simulink model "ARDroneHover"  (R2019a)
settings: Solver=ode1  StartTime=0.0  StopTime=inf  FixedStep=sampleTime  RelTol=1e-3  EnableMultiTasking=on
values from neighbouring files (symbols this model uses):
  choice = input('')    [setupTT.m]
  K = lqr(A,B,Q,R)    [setupTT.m]
  k_w = 1    [setupTT.m]
  sampleTime = 0.03    [setupTT.m]
undefined symbols (not defined in the file or in its folder): DiscIntNeverNeededParam, Standard_Devices, UDP_Protocol
libraries: hdlsllib x6, dspnetwork x4, sldrtlib x3, simulink x1
(part 2 of 2)

== matlab function ARDroneHover/Outer-loop Controller/Error Scopes/normalize angle between -pi and pi radians ==
  data: angleIn input; angleOut output
function angleOut = fcn(angleIn)
%#codegen

angleOut = mod(angleIn, 2*pi) ;
if angleOut > pi
    angleOut = -2*pi + angleOut ; 
end

== matlab function ARDroneHover/Outer-loop Controller/MATLAB Function ==
  data: w_r output; dot_psi_r output; theta_r output; states input; pd input; dot_pd input; ddot_pd input; psi_d input; xi input; phi_r output; dot_xi output; k_w input; K input
function [w_r, dot_psi_r, theta_r, phi_r, dot_xi] = tt_controller(states, pd, dot_pd, ddot_pd,psi_d,xi, k_w, K)
%#codegen

% ------------------------------------------------------------------------
% inputs:
% states - structure with state variables
% pd - desired position
% dot_pd - desired velocity
% ddot_pt - desired acceleration
% psi_d - desired yaw angle
% xi - integral state (four variables)
%
% outputs:
% w_r - vertical velocity reference
% dot_psi_r - yaw rate reference
% theta_r - pitch angle reference
% phi_r - roll angle reference
% dot_xi - integral state derivative
% ------------------------------------------------------------------------

lambda      = states(1:3,1); % Euler angles
psi         = lambda(3);
R           = euler2R(lambda);
Rz          = [cos(psi) -sin(psi) 0; sin(psi) cos(psi) 0; 0 0 1];
psi_e       = normalize_angle(psi-psi_d);

p           = states(7:9,1); % position vector
p(3)        = p(3); % height is symmetric of z
vb          = states(4:6,1); % velocity vector in body coordinates
dot_p       = R*vb; % body velocity rotated to inertial frame 
dot_p(3)    = dot_p(3);

%!!!!!!!!!!!!!!!!!!!!!!!!!!!!!!!!!!!!!!!!!!!!!!!!!!!!!!!!!!!!!!!!!!!!!!
% replace with the necessary code to implement the trajectory tracking
% controller
% pd(3)       = pd(3);
% dot_pd(3)   = dot_pd(3);

% HEIGHT CONTROL
w_r     = -k_w*(p(3) - pd(3));

% OTHER CONTROL
tilde_x     = [p - pd; dot_p - dot_pd];

u_star      = Rz^(-1)*(K*tilde_x + [0; 0; 9.81] - ddot_pd + xi(1:3));

k_w         = 0;
theta_r     = atan(u_star(1)/u_star(3));
phi_r       = atan(-u_star(2)/sqrt(u_star(1)^2+u_star(3)^2));
dot_xi      = [k_w*1*K*tilde_x; psi_e];
dot_xi(3)   = dot_xi(3);

% PSI CONTROL
dot_psi_r   = -1*psi_e - 0.1*xi(4);
%!!!!!!!!!!!!!!!!!!!!!!!!!!!!!!!!!!!!!!!!!!!!!!!!!!!!!!!!!!!!!!!!!!!!!!


function R = euler2R(l)
%#codegen
% returns the rotation matrix for a given vector of euler angles

phi = l(1); theta = l(2); psi = l(3);
R = [cos(theta)*cos(psi)...
      sin(phi)*sin(theta)*cos(psi)-cos(phi)*sin(psi)...
      cos(phi)*sin(theta)*cos(psi)+sin(phi)*sin(psi);
   cos(theta)*sin(psi)...
   sin(phi)*sin(theta)*sin(psi)+cos(phi)*cos(psi)... 
   cos(phi)*sin(theta)*sin(psi)-sin(phi)*cos(psi);
   -sin(theta)...
   sin(phi)*cos(theta)...
   cos(phi)*cos(theta)];

function angleOut = normalize_angle(angleIn)
%#codegen

angleOut = mod(angleIn, 2*pi) ;
if angleOut > pi
    angleOut = -2*pi + angleOut ; 
end

== matlab function ARDroneHover/Data to States/Compute the Derivative/MATLAB Function ==
  data: u input; y output
function y = ZOH_nan(u)

persistent u_

if isempty(u_)
    u_ = 0;
end

if isnan(u)
    u = u_;
else
    u_ = u;
end

y = u;

== matlab function ARDroneHover/Data to States/Compute the Derivative/MATLAB Function1 ==
  data: u input; y output
function y = ZOH_nan(u)

persistent u_

if isempty(u_)
    u_ = 0;
end

if isnan(u)
    u = u_;
else
    u_ = u;
end

y = u;

== matlab function ARDroneHover/Data to States/Compute the Derivative/MATLAB Function2 ==
  data: u input; y output
function y = ZOH_nan(u)

persistent u_

if isempty(u_)
    u_ = 0;
end

if isnan(u)
    u = u_;
else
    u_ = u;
end

y = u;

== matlab function ARDroneHover/Data from Qualisys/Subsystem/MATLAB Function1 ==
  data: x4 output uint8; x3 output uint8; x2 output uint8; data input; x1 output uint8; object input
function [x4,x3,x2,x1] = fcn(data,object)

slot=(object-1)*8;

x1=data(41+slot);
x2=data(41+slot+1);
x3=data(41+slot+2);
x4=data(41+slot+3);

== matlab function ARDroneHover/Data from Qualisys/Subsystem/MATLAB Function2 ==
  data: x input uint32 size=1; X output single size=1; y input; Y output; z input; roll input; pitch input; yaw input; Z output; Roll output; Pitch output; Yaw output
function [X,Y,Z,Roll,Pitch,Yaw] = fcn(x,y,z,roll,pitch,yaw)


X = typecast(uint32(x),'single');
Y = typecast(uint32(y),'single');
Z = typecast(uint32(z),'single');
Roll = typecast(uint32(roll),'single');
Pitch = typecast(uint32(pitch),'single');
Yaw = typecast(uint32(yaw),'single');

== matlab function ARDroneHover/Data from Qualisys/Subsystem/MATLAB Function3 ==
  data: y4 output uint8; y3 output uint8; y2 output uint8; data input; y1 output uint8; object input
function [y4,y3,y2,y1] = fcn(data,object)

slot=(object-1)*8;

y1=data(45+slot);
y2=data(45+slot+1);
y3=data(45+slot+2);
y4=data(45+slot+3);

== matlab function ARDroneHover/Data from Qualisys/Subsystem/MATLAB Function4 ==
  data: z4 output uint8; z3 output uint8; z2 output uint8; data input; z1 output uint8; object input
function [z4,z3,z2,z1] = fcn(data,object)

slot=(object-1)*8;

z1=data(49+slot);
z2=data(49+slot+1);
z3=data(49+slot+2);
z4=data(49+slot+3);

== matlab function ARDroneHover/Data from Qualisys/Subsystem/MATLAB Function5 ==
  data: roll4 output uint8; roll3 output uint8; roll2 output uint8; data input; roll1 output uint8; object input
function [roll4,roll3,roll2,roll1] = fcn(data,object)

slot=(object-1)*8;

roll1=data(53+slot);
roll2=data(53+slot+1);
roll3=data(53+slot+2);
roll4=data(53+slot+3);

== matlab function ARDroneHover/Data from Qualisys/Subsystem/MATLAB Function6 ==
  data: pitch4 output uint8; pitch3 output uint8; pitch2 output uint8; data input; pitch1 output uint8; object input
function [pitch4,pitch3,pitch2,pitch1] = fcn(data,object)

slot=(object-1)*8;

pitch1=data(57+slot);
pitch2=data(57+slot+1);
pitch3=data(57+slot+2);
pitch4=data(57+slot+3);

== matlab function ARDroneHover/Data from Qualisys/Subsystem/MATLAB Function7 ==
  data: yaw4 output uint8; yaw3 output uint8; yaw2 output uint8; data input; yaw1 output uint8; object input
function [yaw4,yaw3,yaw2,yaw1] = fcn(data,object)

slot=(object-1)*8;

yaw1=data(61+slot);
yaw2=data(61+slot+1);
yaw3=data(61+slot+2);
yaw4=data(61+slot+3);

== matlab function ARDroneHover/Data to States/MATLAB Function ==
  data: v input; v_b output; phi input; theta input; psi input
function v_b = fcn(v,phi,theta,psi)

R = [cos(theta)*cos(psi)...
      sin(phi)*sin(theta)*cos(psi)-cos(phi)*sin(psi)...
      cos(phi)*sin(theta)*cos(psi)+sin(phi)*sin(psi);
   cos(theta)*sin(psi)...
   sin(phi)*sin(theta)*sin(psi)+cos(phi)*cos(psi)... 
   cos(phi)*sin(theta)*sin(psi)-sin(phi)*cos(psi);
   -sin(theta)...
   sin(phi)*cos(theta)...
   cos(phi)*cos(theta)];

v_b = R'*v;

== matlab function ARDroneHover/MATLAB Function1 ==
  data: on_off input; states input; t input; pd output; dot_pd output; ddot_pd output; psi_d output; choice input
function [pd, dot_pd, ddot_pd, psi_d] = desired_trajectory(on_off,states,t, choice)
%#codegen

% ------------------------------------------------------------------------
% inputs:
% on_off - 1 if tracking is on, 0 if it is off
% states - structure with state variables
% t - current simulation time
% 
% outputs:
% pd - desired position
% dot_pd - desired velocity
% ddot_pd - desired acceleration
% psi_d - desired yaw angle
% ------------------------------------------------------------------------

persistent t0
persistent p0
persistent previous_status

on  = 1;
off = 0;

BASE_ALT = 1;

% RESETS THE 0
if isempty(previous_status)
    previous_status = on;
    p0 = [states(7:8);BASE_ALT];
end

if on_off == off
    if previous_status == on 
    % first time off or switching back off
        p0 = [states(7:8);BASE_ALT]; % x0 and y0 match the current position
    end
    pd = p0;
    dot_pd = [0;0;0];
    ddot_pd = [0;0;0];
    psi_d = 0;
else
    if isempty(t0) || (previous_status == off) 
    % first time on or switching back on
        t0 = t;
        p0 = [states(7:8);BASE_ALT];
    end
    dt = t-t0;

%!!!!!!!!!!!!!!!!!!!!!!!!!!!!!!!!!!!!!!!!!!!!!!!!!!!!!!!!!!!!!!!!!!!!!!!!
% replace with the necessary code to define adequate desired trajectories
% use dt, p0, and any additional parameters

pd      = p0;
t_init  = 10;
t_track = 20;

% DEFINES THE STARTING HEIGHT
if(dt > t_init)
    pd(3) = pd(3) + 0.25;  
else
    pd(3) = pd(3) + 0;  
end

% DIFFERENT TRACKS
switch choice
    %--- Altitude Tracking ---
    case 1
      dot_pd    = [0;0;0];
      ddot_pd   = [0;0;0];
      psi_d     = 0;
    % --- Horizontal Line in X-Y ---
    case 2
      ang = 45;
      vel = 0.5;

      if(dt > t_track)
        dot_pd  = [vel*cosd(ang); vel*sind(ang);0];
        pd(1)   = p0(1) + vel*cosd(ang)*(dt - t_track);
        pd(2)   = p0(2) + vel*sind(ang)*(dt - t_track);
      else
        dot_pd  = [0;0;0]; 
      end
      
      ddot_pd   = [0;0;0];
      psi_d     = 0;
    % --- Circular Line - Constant Yaw ---
	case 3
      ang_rate = 0.1; %rad/s

      if(dt > t_track)
        pd(1:2)	= [ cos(ang_rate*(dt - t_track)) - 1;... 
                    sin(ang_rate*(dt - t_track))];
        dot_pd	= [-sin(ang_rate*(dt - t_track));...
                    cos(ang_rate*(dt - t_track));0]*ang_rate;
        ddot_pd = [-cos(ang_rate*(dt - t_track));...
                   -sin(ang_rate*(dt - t_track));0]*(ang_rate^2);
      else
        dot_pd  = [0;0;0]; 
        ddot_pd = [0;0;0]; 
      end
      psi_d = 0;
    % --- Circular Line - Variable Yaw ---
    case 4
      ang_rate  = 0.1; %rad/s
      R         = 1;
      if(dt > t_track)
        pd(1:2)	= [ cos(ang_rate*(dt - t_track)) - 1;... 
                    sin(ang_rate*(dt - t_track))  ]*R;
        dot_pd	= [-sin(ang_rate*(dt - t_track));...
                    cos(ang_rate*(dt - t_track));0]*R*ang_rate;
        ddot_pd = [-cos(ang_rate*(dt - t_track));...
                   -sin(ang_rate*(dt - t_track));0]*R*(ang_rate^2);
        %psi_d = pi/2;
        psi_d   =       ang_rate*(dt - t_track);
      else
        dot_pd  = [0;0;0]; 
        ddot_pd = [0;0;0];
        psi_d   = 0;
      end
    % --- Line of Sight ---
    case 5
      Delta  = 0.3; 
      V      = 0.1;
      yd     = p0(2) + 1;
      %vel = 0.1;
      if(dt > t_track)
        %pd(1:2)	= p0(1:2) + [V*(dt - t_track); 1];
        pd(1:2)   = states(7:8);
        psi_d     = atan(-(states(8) - yd)/Delta);
        dot_pd	  = [cos(psi_d);sin(psi_d);0]*V;
        %ddot_pd   = [0;0;0];
        dot_psi_d = (-states(5)/Delta)/(1+(-(states(8)-yd)/Delta)^2);
        ddot_pd   = [-V*dot_psi_d*sin(psi_d); V*dot_psi_d*cos(psi_d); 0];
      else
        dot_pd  = [0;0;0]; 
        ddot_pd = [0;0;0];
        psi_d   = 0;
      end  
    otherwise
      pd        = p0;
      dot_pd    = [0;0;0];
      ddot_pd   = [0;0;0];
      psi_d     = 0;
end
        
%!!!!!!!!!!!!!!!!!!!!!!!!!!!!!!!!!!!!!!!!!!!!!!!!!!!!!!!!!!!!!!!!!!!!!!!!

end

previous_status = on_off;
